simulink model "LQR_control_AND_Plant30April2026"  (R2022a)
settings: Solver=VariableStepAuto  StartTime=0.0  StopTime=10.0  RelTol=1e-3
values from neighbouring files (symbols this model uses):
  K = lqr(A_Mat, B_Mat, Q, R)    [LQR_code.m]
settings Model: Creator=Mahmoud Essam  LastModifiedBy=Electronica Care
settings ModelReferenceCC: EnableRefExpFcnMdlSchedulingChecks=off
settings RTWCC: Description=Generic Real-Time Target  GPUComputeCapability=5.0

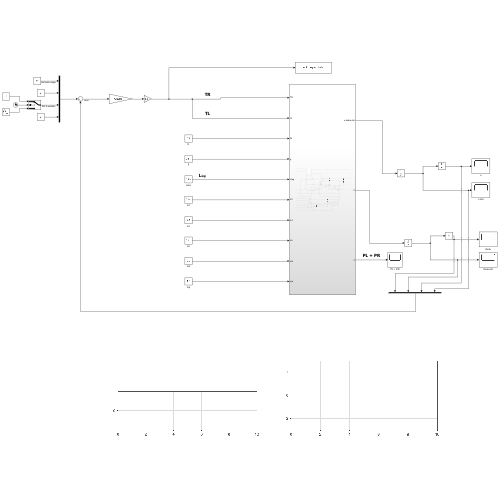
[thumbnail: Simulink's stored preview of the top-level diagram]
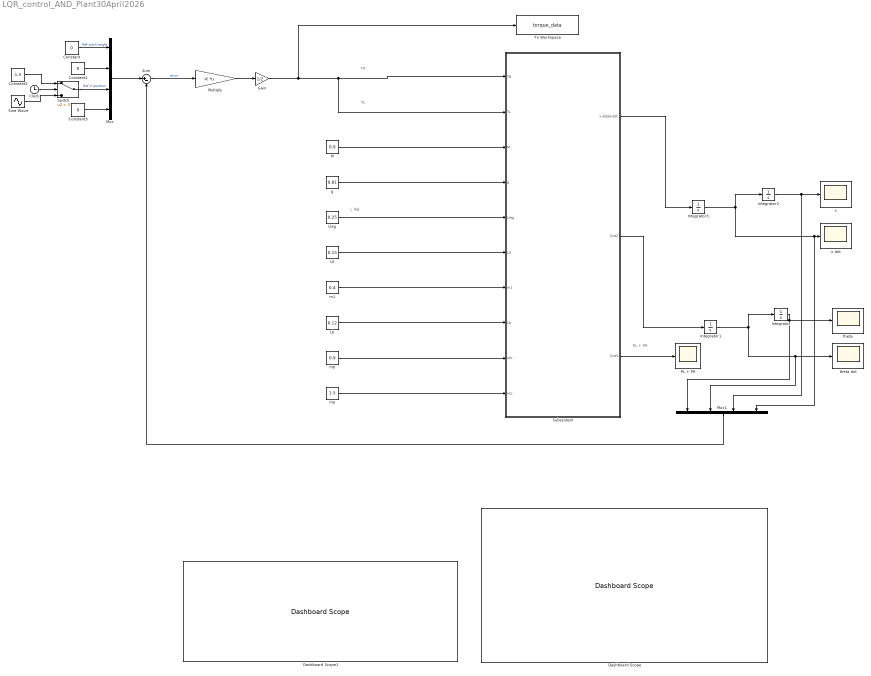
== system LQR_control_AND_Plant30April2026 ==
  note: TR
  note: L leg
  note: PL + PR
  note: TL
  Clock : Clock
  Constant : Constant  Value=0
  Constant1 : Constant  Value=0
  Constant2 : Constant  Value=1.5
  Constant3 : Constant  Value=0
  Dashboard Scope : DashboardScope
  Dashboard Scope1 : DashboardScope
  Gain : Gain  Gain=1/2
  Integrator{,1..3} (4 alike) : Integrator
  L0 : Constant  Value=0.15
  Lb : Constant  Value=0.12
  Lleg : Constant  Value=0.25
  M : Constant  Value=0.9
  Multiply : Gain  Gain=-K  Multiplication=Matrix(K*u) (u vector)
  Mux : Mux
  Mux1 : Mux
  PL + PR : Scope
  Sine Wave : Sin  Amplitude=1.5  Frequency=.5  SampleTime=0
  Subsystem : Subsystem
  Sum : Sum  Inputs=|+-
  Switch : Switch  Criteria=u2 > Threshold  Threshold=3  SaturateOnIntegerOverflow=off  InputSameDT=off
  To Workspace : ToWorkspace  VariableName=torque_data  SampleTime=-1
  g : Constant  Value=9.81
  m1 : Constant  Value=0.4
  mb : Constant  Value=0.9
  mp : Constant  Value=1.5
  theta : Scope
  theta dot : Scope
  x : Scope
  x dot : Scope
  wires:
  Multiply/1 -> Gain/1
  Sum/1 -> Multiply/1  "error"
  Mux/1 -> Sum/1
  Constant3/1 -> Mux/4
  Switch/1 -> Mux/3  "Ref X position"
  Constant1/1 -> Mux/2
  Constant/1 -> Mux/1  "Ref pitch angle"
  Clock/1 -> Switch/2
  Sine Wave/1 -> Switch/3
  Constant2/1 -> Switch/1
  Integrator1/1 -> Mux1/2, theta dot/1, Integrator/1
  Integrator/1 -> theta/1, Mux1/1
  Subsystem/3(Out3) -> PL + PR/1
  Subsystem/2(Out2) -> Integrator1/1
  m1/1 -> Subsystem/7(m1)
  g/1 -> Subsystem/4(g)
  M/1 -> Subsystem/3(M)
  L0/1 -> Subsystem/6(L0)
  Lleg/1 -> Subsystem/5(Lleg)
  mb/1 -> Subsystem/9(mb)
  Gain/1 -> To Workspace/1, Subsystem/2(TL), Subsystem/1(TR)
  mp/1 -> Subsystem/10(mp)
  Lb/1 -> Subsystem/8(Lb)
  Integrator2/1 -> x/1, Mux1/3
  Integrator3/1 -> x dot/1, Mux1/4, Integrator2/1
  Subsystem/1(x duble dot) -> Integrator3/1
  Mux1/1 -> Sum/2

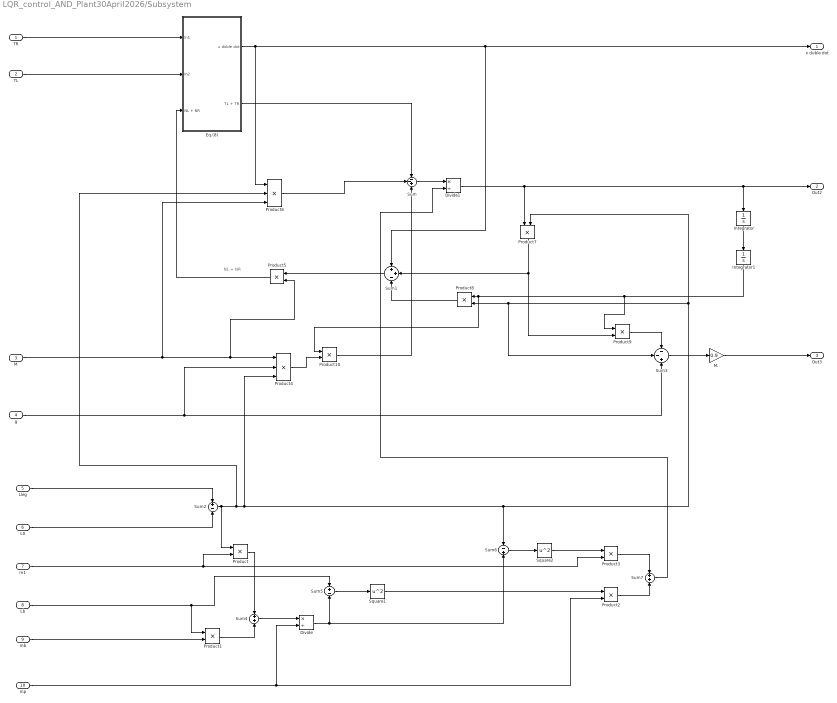
== system LQR_control_AND_Plant30April2026/Subsystem ==
  note: NL + NR
  TR : Inport
  TL : Inport  Port=2
  M : Inport  Port=3
  g : Inport  Port=4
  Lleg : Inport  Port=5
  L0 : Inport  Port=6
  m1 : Inport  Port=7
  Lb : Inport  Port=8
  mb : Inport  Port=9
  mp : Inport  Port=10
  Divide : Product  Inputs=*/
  Divide1 : Product  Inputs=*/
  Eq.(8) : Subsystem
  Integrator : Integrator
  Integrator1 : Integrator
  M. : Gain  Gain=0.9
  Product{,1..3,5,7..10} (9 alike) : Product
  Product4 : Product  Inputs=3
  Product6 : Product  Inputs=3
  Square1 : Math  Operator=square
  Square2 : Math  Operator=square
  Sum : Sum  Inputs=--+
  Sum1 : Sum  Inputs=++-
  Sum2 : Sum  Inputs=+-
  Sum3 : Sum  Inputs=--+
  Sum4 : Sum
  Sum5 : Sum  Inputs=+-
  Sum6 : Sum  Inputs=-+
  Sum7 : Sum
  x duble dot : Outport
  Out2 : Outport  Port=2
  Out3 : Outport  Port=3
  wires:
  Eq.(8)/2(TL + TR) -> Sum/1
  Product3/1 -> Sum7/1
  Square2/1 -> Product3/1
  Eq.(8)/1(x duble dot) -> x duble dot/1, Sum1/1, Product6/1
  M./1 -> Out3/1
  Product9/1 -> Sum3/1
  Product8/1 -> Sum1/3
  g/1 -> Sum3/3, Product4/2
  m1/1 -> Product3/2, Product/2
  Sum/1 -> Divide1/1
  Product6/1 -> Sum/2
  Sum2/1 -> Product6/2, Sum6/1, Product8/2, Sum3/2, Product7/2, Product4/3, Product/1
  Sum5/1 -> Square1/1
  Sum3/1 -> M./1
  mb/1 -> Product1/2
  Product4/1 -> Product10/2
  Divide1/1 -> Product7/1, Out2/1, Integrator/1
  M/1 -> Product4/1, Product5/2, Product6/3
  Divide/1 -> Sum5/2, Sum6/2
  Sum7/1 -> Divide1/2
  Product2/1 -> Sum7/2
  TL/1 -> Eq.(8)/2(In2)
  Product7/1 -> Product9/2, Sum1/2
  Product5/1 -> Eq.(8)/3(NL + NR)
  Sum1/1 -> Product5/1
  Product/1 -> Sum4/1
  Product1/1 -> Sum4/2
  Square1/1 -> Product2/1
  Sum6/1 -> Square2/1
  mp/1 -> Product2/2, Divide/2
  Sum4/1 -> Divide/1
  Product10/1 -> Sum/3
  Lb/1 -> Sum5/1, Product1/1
  Lleg/1 -> Sum2/1
  TR/1 -> Eq.(8)/1(In1)
  L0/1 -> Sum2/2
  Integrator/1 -> Integrator1/1
  Integrator1/1 -> Product9/1, Product10/1, Product8/1

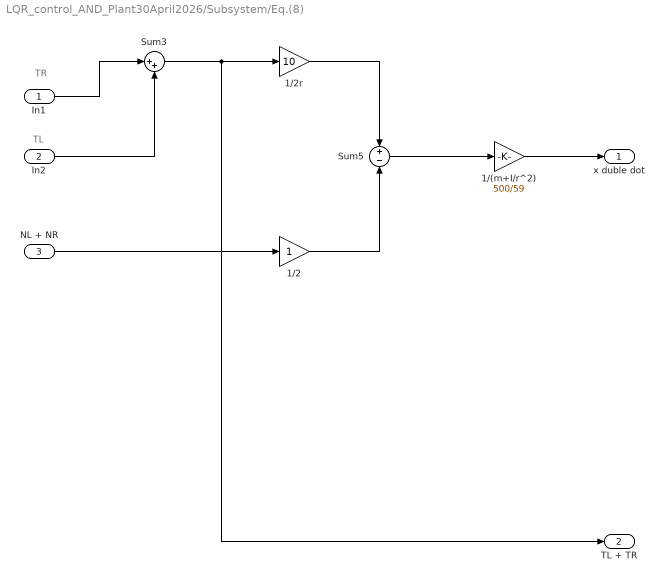
== system LQR_control_AND_Plant30April2026/Subsystem/Eq.(8) ==
  note: TL
  note: TR
  In1 : Inport
  In2 : Inport  Port=2
  NL + NR : Inport  Port=3
  1/(m+I/r^2) : Gain  Gain=500/59
  1/2 : Gain
  1/2r : Gain  Gain=10
  Sum3 : Sum  Inputs=|++
  Sum5 : Sum  Inputs=+-
  x duble dot : Outport
  TL + TR : Outport  Port=2
  wires:
  In1/1 -> Sum3/1
  In2/1 -> Sum3/2
  1/2/1 -> Sum5/2
  1/2r/1 -> Sum5/1
  NL + NR/1 -> 1/2/1
  Sum3/1 -> TL + TR/1, 1/2r/1
  Sum5/1 -> 1/(m+I/r^2)/1
  1/(m+I/r^2)/1 -> x duble dot/1
